simulink library "SecureTElib"  (R2017a)
settings: Solver=VariableStepAuto  StartTime=0.0  StopTime=10.0  RelTol=1e-3
settings Model: Creator=ryuga  LastModifiedBy=ryuga

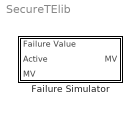
== system SecureTElib ==
  Failure Simulator : Subsystem

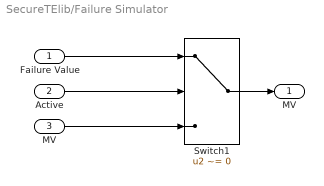
== system SecureTElib/Failure Simulator ==
  Failure Value : Inport
  "Active " : Inport  Port=2
  MV : Inport  Port=3
  Switch1 : Switch  Criteria=u2 ~= 0
  "MV " : Outport
  wires:
  "Active "/1 -> Switch1/2
  MV/1 -> Switch1/3
  Failure Value/1 -> Switch1/1
  Switch1/1 -> "MV "/1
